simulink model "six_plus_six_AcmsteeringV09_main"  (R2014a)
settings: Solver=FixedStepDiscrete  StartTime=0.0  StopTime=10.0  FixedStep=0.0005  RelTol=1e-3
InitFcn:
  | Veh_Par_wxt
values from neighbouring files (symbols this model uses):
  acc_spdctl = [0 100]    [Veh_Par_wxt.m]
  ag_thr = ecucoder_cal(ag_thr)    [Veh_Par_wxt.m]
  B = 1.8    [Veh_Par_wxt.m]
  bra_em = 100    [Veh_Par_wxt.m]
  bra_pre_gz2 = 100/3    (= 33.3333333333)    [Veh_Par_wxt.m]
  bra_pre_gz34 = 10/3    (= 3.33333333333)    [Veh_Par_wxt.m]
  bra_pre_yd = 10/2    (= 5)    [Veh_Par_wxt.m]
  brakepre_dem_data = [0 1 2 3 4 5 6 7 8 9 10]    [Veh_Par_wxt.m]
  brakeTrq_dem_data = [0 125 251 376 502 627 753 878 1004 1129 1255]    [Veh_Par_wxt.m]
  bratrq_max = 4*1255    (= 5020)    [Veh_Par_wxt.m]
  eff_tran = 0.9    [Veh_Par_wxt.m]
  ESP_switch = ecucoder_cal(ESP_switch)    [Veh_Par_wxt.m]
  G = Mass*g    (= 15696)    [Veh_Par_wxt.m]
  kd1 = ecucoder_cal(kd1)    [Veh_Par_wxt.m]
  kd2 = 0    [Veh_Par_wxt.m]
  ki1 = ecucoder_cal(ki1)    [Veh_Par_wxt.m]
  ki2 = 1    [Veh_Par_wxt.m]
  kp1 = ecucoder_cal(kp1)    [Veh_Par_wxt.m]
  kp2 = 300    [Veh_Par_wxt.m]
  L = L1+L2    (= 2.9)    [Veh_Par_wxt.m]
  premax = 100    [Veh_Par_wxt.m]
  Radius = 0.4572/2    (= 0.2286)    [Veh_Par_wxt.m]
  RC_switch = ecucoder_cal(RC_switch)    [Veh_Par_wxt.m]
  s_opt_yi = 0.15    [Veh_Par_wxt.m]
  s_opt_zhuan = 0.8    [Veh_Par_wxt.m]
  s_opt_zhuan_add = 0.05    [Veh_Par_wxt.m]
  s_opt_zhuan_table = [0.8 0.8 0.3 0.3]    [Veh_Par_wxt.m]
  spd_map_mot = [0 499.85 999.79 1500 2000 2500 3000 3500 4000 4500 4999.8 5999.8]    [Veh_Par_wxt.m]
  spd_spdctl = [0 500]    [Veh_Par_wxt.m]
  speed_thr_park = 5/3.6/Radius*tras_ratio*30/pi    (= 464.143899364)    [Veh_Par_wxt.m]
  TCS_switch = ecucoder_cal(TCS_switch)    [Veh_Par_wxt.m]
  tras_ratio = 8    [Veh_Par_wxt.m]
  trq_map_mot = [70.5 70.012 71.154 65.797 53.917 45.159 38.073 32.685 27.48 17.133 14.949 10.07]    [Veh_Par_wxt.m]
  trqmax_yd = 70.5    [Veh_Par_wxt.m]
  trqmax_zx = 70.5    [Veh_Par_wxt.m]
  trqmaxneg = -70.5    [Veh_Par_wxt.m]
  v_gain = 0.9    [Veh_Par_wxt.m]
  v_table = [0 5 20 100]    [Veh_Par_wxt.m]
  v_thr_park = 5    [Veh_Par_wxt.m]
  zhidong_bianmazhi = [-140000 750000]    [Veh_Par_wxt.m]
  zhidong_down = -140000    [Veh_Par_wxt.m]
  zhidong_up = 750000    [Veh_Par_wxt.m]
  zhidong_youmen = [0 100]    [Veh_Par_wxt.m]
  zhuanxiang_bianmazhi = [-400000 0 400000]    [Veh_Par_wxt.m]
  zhuanxiang_down = -400000    [Veh_Par_wxt.m]
  zhuanxiang_up = 400000    [Veh_Par_wxt.m]
  zhuanxiang_youmen = [-100 0 100]    [Veh_Par_wxt.m]
undefined symbols (not defined in the file or in its folder): ecucoder_acal, guzhang_lf, guzhang_lm, guzhang_lr, guzhang_rf, guzhang_rm, guzhang_rr, myFIS
libraries: simulink x979, ec5744lib x59, fuzblock x2
(part 25 of 26)

== system six_plus_six_AcmsteeringV09_main/MainControl/mode_control/forward/forward/Drive/驱动防滑控制TCS/直行TCS/Subsystem5 ==
  speed_act_rr : Inport
  v_act : Inport  Port=2
  Add : Sum
  Constant : Constant  Value=eps  OutDataTypeStr=single  SampleTime=-1
  Divide : Product  Inputs=*/
  Gain : Gain  Gain=pi/30
  Gain1 : Gain  Gain=Radius
  Gain2 : Gain  Gain=1/3.6
  Gain3 : Gain  Gain=1/tras_ratio
  Subtract : Sum  Inputs=+-
  s_act_rr : Outport
  wires:
  Divide/1 -> s_act_rr/1
  Add/1 -> Divide/2
  Constant/1 -> Add/2
  Subtract/1 -> Divide/1
  Gain1/1 -> Subtract/1, Add/1
  v_act/1 -> Gain2/1
  Gain/1 -> Gain1/1
  speed_act_rr/1 -> Gain3/1
  Gain3/1 -> Gain/1
  Gain2/1 -> Subtract/2

== system six_plus_six_AcmsteeringV09_main/MainControl/mode_control/forward/forward/Drive/驱动防滑控制TCS/直行TCS/Subsystem6 ==
  speed_act_lf : Inport
  speed_act_lm : Inport  Port=2
  speed_act_lr : Inport  Port=3
  Gain : Gain  Gain=1/tras_ratio
  Gain1 : Gain  Gain=pi/30
  Gain2 : Gain  Gain=Radius
  Gain3 : Gain  Gain=3.6
  Gain4 : Gain  Gain=v_gain
  MinMax : MinMax  Inputs=3
  v_act_l : Outport
  wires:
  speed_act_lm/1 -> MinMax/2
  speed_act_lr/1 -> MinMax/3
  speed_act_lf/1 -> MinMax/1
  MinMax/1 -> Gain/1
  Gain/1 -> Gain1/1
  Gain1/1 -> Gain2/1
  Gain2/1 -> Gain3/1
  Gain3/1 -> Gain4/1
  Gain4/1 -> v_act_l/1

== system six_plus_six_AcmsteeringV09_main/MainControl/mode_control/forward/forward/Drive/驱动防滑控制TCS/直行TCS/Subsystem7 ==
  speed_act_rf : Inport
  speed_act_rm : Inport  Port=2
  speed_act_rr : Inport  Port=3
  Gain : Gain  Gain=1/tras_ratio
  Gain1 : Gain  Gain=pi/30
  Gain2 : Gain  Gain=Radius
  Gain3 : Gain  Gain=3.6
  Gain4 : Gain  Gain=v_gain
  MinMax : MinMax  Inputs=3
  v_act_r : Outport
  wires:
  Gain4/1 -> v_act_r/1
  Gain3/1 -> Gain4/1
  Gain2/1 -> Gain3/1
  Gain1/1 -> Gain2/1
  Gain/1 -> Gain1/1
  MinMax/1 -> Gain/1
  speed_act_rf/1 -> MinMax/1
  speed_act_rr/1 -> MinMax/3
  speed_act_rm/1 -> MinMax/2

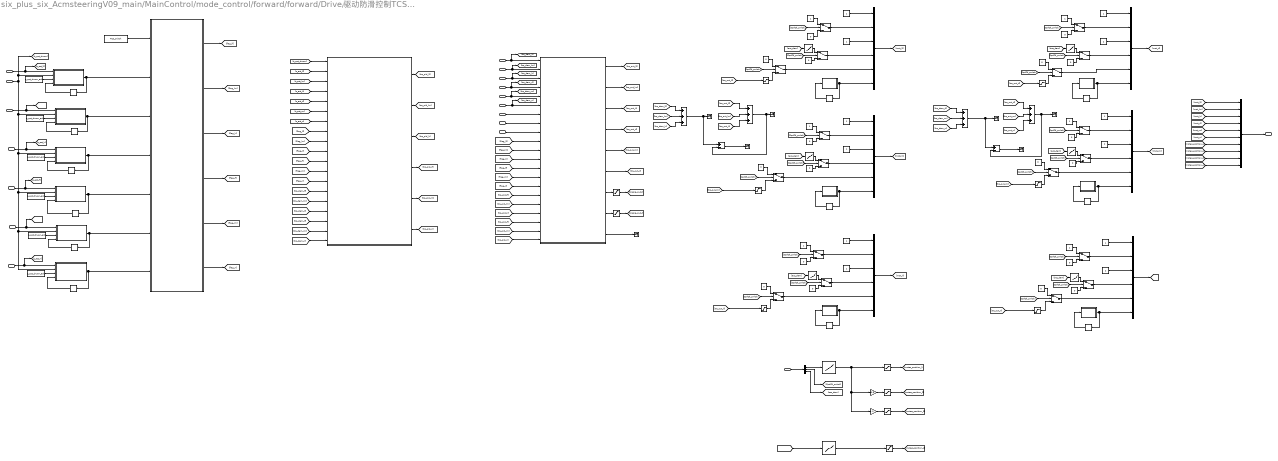
== system six_plus_six_AcmsteeringV09_main/MainControl/mode_control/forward/forward/Drive/驱动防滑控制TCS/直行TCS/直行 ==
  trq_dem_lf : Inport
  trq_dem_lm : Inport  Port=2
  trq_dem_lr : Inport  Port=3
  trq_dem_rf : Inport  Port=4
  trq_dem_rm : Inport  Port=5
  trq_dem_rr : Inport  Port=6
  bra_pre_l : Inport  Port=7
  bra_pre_r : Inport  Port=8
  s_act_lf : Inport  Port=9
  s_act_lm : Inport  Port=10
  s_act_lr : Inport  Port=11
  s_act_rf : Inport  Port=12
  s_act_rm : Inport  Port=13
  s_act_rr : Inport  Port=14
  brake_dem : Inport  Port=15
  s_opt_zhuan : Inport  Port=16
  Signals : Inport  Port=17
  1-D Lookup Table : Lookup_n-D  NumberOfTableDimensions=1  BreakpointsForDimension1=zhuanxiang_youmen  Table=zhuanxiang_bianmazhi  InternalRulePriority=Speed  RndMeth=Simplest  InputSameDT=on
  1-D Lookup Table1 : Lookup_n-D  NumberOfTableDimensions=1  BreakpointsForDimension1=zhidong_youmen  Table=zhidong_bianmazhi  InternalRulePriority=Speed  RndMeth=Simplest  InputSameDT=on
  1-D Lookup Table{2..7} (6 alike) : Lookup_n-D  NumberOfTableDimensions=1  BreakpointsForDimension1=acc_spdctl  Table=spd_spdctl  InternalRulePriority=Speed  RndMeth=Simplest  InputSameDT=on
  Add{,1..3} (4 alike) : Sum  Inputs=+++
  Bus Selector : BusSelector  OutputSignals=RemoteControl_dem.steer_dem,RemoteControl_dem.SpdCtl_switch,RemoteControl_dem.acc_dem
  Constant{,1,3..6} (6 alike) : Constant  Value=0  OutDataTypeStr=single  SampleTime=-1
  Constant{7..10,12..13} (6 alike) : Constant  Value=s_opt_zhuan_add  OutDataTypeStr=single  SampleTime=-1
  Constant11 : Constant  Value=TCS_switch  OutDataTypeStr=single  SampleTime=-1
  Gain : Gain  Gain=0.5
  Gain1 : Gain  Gain=-1
  HeartBeat : MATLAB Function  TreatAsAtomicUnit=on
  HeartBeat1 : MATLAB Function  TreatAsAtomicUnit=on
  HeartBeat2 : MATLAB Function  TreatAsAtomicUnit=on
  HeartBeat3 : MATLAB Function  TreatAsAtomicUnit=on
  HeartBeat4 : MATLAB Function  TreatAsAtomicUnit=on
  HeartBeat5 : MATLAB Function  TreatAsAtomicUnit=on
  MATLAB Function : MATLAB Function  TreatAsAtomicUnit=on
  MATLAB Function1 : MATLAB Function  TreatAsAtomicUnit=on
  MATLAB Function2 : MATLAB Function  TreatAsAtomicUnit=on
  MATLAB Function3 : MATLAB Function  TreatAsAtomicUnit=on
  MATLAB Function4 : MATLAB Function  TreatAsAtomicUnit=on
  MATLAB Function5 : MATLAB Function  TreatAsAtomicUnit=on
  MATLAB Function6 : MATLAB Function  TreatAsAtomicUnit=on
  MATLAB Function7 : MATLAB Function  TreatAsAtomicUnit=on
  Memory{,1..11} (12 alike) : Memory  InheritSampleTime=on
  Mux : Mux  Inputs=10
  Mux{1..6} (6 alike) : Mux  Inputs=6
  Saturation{,1..3,6..7} (6 alike) : Saturate  UpperLimit=trqmax_zx  LowerLimit=trqmaxneg  OutDataTypeStr=single
  Saturation10 : Saturate  UpperLimit=zhuanxiang_up  LowerLimit=zhuanxiang_down
  Saturation11 : Saturate  UpperLimit=zhidong_up  LowerLimit=zhidong_down
  Saturation4 : Saturate  UpperLimit=premax  LowerLimit=0
  Saturation5 : Saturate  UpperLimit=premax  LowerLimit=0
  Saturation8 : Saturate  UpperLimit=zhuanxiang_up  LowerLimit=zhuanxiang_down
  Saturation9 : Saturate  UpperLimit=zhuanxiang_up  LowerLimit=zhuanxiang_down
  SpdSet_dem{,1..5} (6 alike) : Constant  Value=0  OutDataTypeStr=single  SampleTime=-1
  Subsystem : Subsystem
  Subtract : Sum  Inputs=+-
  Subtract1 : Sum  Inputs=+-
  Switch{,1..17} (18 alike) : Switch  Criteria=u2 > Threshold  Threshold=0.5
  Terminator{1..7} (7 alike) : Terminator
  mot_enable{1..6} (6 alike) : Constant  OutDataTypeStr=single  SampleTime=-1
  mot_gear : Constant  OutDataTypeStr=single  SampleTime=-1
  mot_gear1 : Constant  Value=2  OutDataTypeStr=single  SampleTime=-1
  mot_gear2 : Constant  OutDataTypeStr=single  SampleTime=-1
  mot_gear3 : Constant  Value=2  OutDataTypeStr=single  SampleTime=-1
  mot_gear4 : Constant  OutDataTypeStr=single  SampleTime=-1
  mot_gear5 : Constant  Value=2  OutDataTypeStr=single  SampleTime=-1
  mot_mode{,1..5} (6 alike) : Constant  Value=0  OutDataTypeStr=single  SampleTime=-1
  mot_mode{6..11} (6 alike) : Constant  OutDataTypeStr=single  SampleTime=-1
  forward_dem : Outport
  wires:
  Mux/1 -> forward_dem/1
  Memory4/1 -> HeartBeat/1(life_pre)
  HeartBeat/1(life) -> Memory4/1, Mux1/6
  Mux1/1 -> [mot_lf]
  [trq_out_lf] -> Saturation/1  "trq_out_lf_forward"
  mot_gear/1 -> Mux1/3
  mot_enable4/1 -> Mux1/1
  Switch1/1 -> Mux1/4
  Memory1/1 -> HeartBeat2/1(life_pre)
  HeartBeat2/1(life) -> Mux3/6, Memory1/1
  Mux3/1 -> [mot_rf]
  [trq_out_rf] -> Saturation2/1  "trq_out_rf_forward"
  Switch3/1 -> Mux3/2
  mot_gear1/1 -> Mux3/3
  mot_enable2/1 -> Mux3/1
  Switch8/1 -> Mux3/4
  Memory2/1 -> HeartBeat3/1(life_pre)
  HeartBeat3/1(life) -> Mux5/6, Memory2/1
  Mux5/1 -> [mot_lm]
  [trq_out_lm] -> Saturation6/1  "trq_out_lm_forward"
  Switch4/1 -> Mux5/2
  mot_gear2/1 -> Mux5/3
  mot_enable5/1 -> Mux5/1
  Switch10/1 -> Mux5/4
  Memory3/1 -> HeartBeat4/1(life_pre)
  HeartBeat4/1(life) -> Memory3/1, Mux6/6
  Mux6/1 -> [mot_rm]
  [trq_out_rm] -> Saturation7/1  "trq_out_rm_forward"
  Switch5/1 -> Mux6/2
  mot_gear3/1 -> Mux6/3
  mot_enable6/1 -> Mux6/1
  Switch11/1 -> Mux6/4
  Memory5/1 -> HeartBeat1/1(life_pre)
  HeartBeat1/1(life) -> Mux2/6, Memory5/1
  Mux2/1 -> [mot_lr]
  [trq_out_lr] -> Saturation1/1  "trq_out_lr_forward"
  Switch6/1 -> Mux2/2
  mot_gear4/1 -> Mux2/3
  mot_enable1/1 -> Mux2/1
  Switch12/1 -> Mux2/4
  Memory6/1 -> HeartBeat5/1(life_pre)
  HeartBeat5/1(life) -> Memory6/1, Mux4/6
  Mux4/1 -> [mot_rr]
  [trq_out_rr] -> Saturation3/1  "trq_out_rr_forward"
  Switch7/1 -> Mux4/2
  mot_gear5/1 -> Mux4/3
  mot_enable3/1 -> Mux4/1
  Switch13/1 -> Mux4/4
  [mot_lf] -> Mux/1
  [mot_lm] -> Mux/2
  [mot_lr] -> Mux/3
  [mot_rf] -> Mux/4
  [mot_rm] -> Mux/5
  [mot_rr] -> Mux/6
  [motec_position_1] -> Mux/7
  [motec_position_2] -> Mux/8
  [motec_position_3] -> Mux/9
  1-D Lookup Table1/1 -> Saturation11/1
  1-D Lookup Table/1 -> Gain1/1, Gain/1, Saturation8/1
  Signals/1 -> Bus Selector/1
  Gain1/1 -> Saturation10/1
  Bus Selector/1 -> 1-D Lookup Table/1  "<steer_dem>"
  Gain/1 -> Saturation9/1
  Saturation8/1 -> [motec_position_1]
  Saturation9/1 -> [motec_position_2]
  Saturation10/1 -> [motec_position_3]
  Saturation11/1 -> [motec_position_4]
  [brapre_out_l] -> 1-D Lookup Table1/1
  [motec_position_4] -> Mux/10
  Bus Selector/2 -> [SpdCtl_switch]  "<SpdCtl_switch>"
  [SpdCtl_switch] -> Switch/2
  mot_mode6/1 -> Switch/1
  mot_mode/1 -> Switch/3
  Switch/1 -> Mux1/2
  [SpdCtl_switch] -> Switch1/2
  SpdSet_dem/1 -> Switch1/3
  Bus Selector/3 -> [acc_dem]  "<acc_dem>"
  [acc_dem] -> 1-D Lookup Table2/1
  1-D Lookup Table2/1 -> Switch1/1
  [SpdCtl_switch] -> Switch2/2
  Saturation/1 -> Switch2/3
  Constant/1 -> Switch2/1
  Switch2/1 -> Mux1/5
  [SpdCtl_switch] -> Switch3/2
  mot_mode7/1 -> Switch3/1
  mot_mode2/1 -> Switch3/3
  [SpdCtl_switch] -> Switch4/2
  mot_mode8/1 -> Switch4/1
  mot_mode4/1 -> Switch4/3
  [SpdCtl_switch] -> Switch5/2
  mot_mode9/1 -> Switch5/1
  mot_mode5/1 -> Switch5/3
  [SpdCtl_switch] -> Switch6/2
  mot_mode10/1 -> Switch6/1
  mot_mode1/1 -> Switch6/3
  [SpdCtl_switch] -> Switch7/2
  mot_mode11/1 -> Switch7/1
  mot_mode3/1 -> Switch7/3
  [SpdCtl_switch] -> Switch8/2
  [acc_dem] -> 1-D Lookup Table3/1
  1-D Lookup Table3/1 -> Switch8/1
  SpdSet_dem1/1 -> Switch8/3
  [SpdCtl_switch] -> Switch9/2
  Constant1/1 -> Switch9/1
  Saturation2/1 -> Switch9/3
  Switch9/1 -> Mux3/5
  [SpdCtl_switch] -> Switch10/2
  [acc_dem] -> 1-D Lookup Table4/1
  1-D Lookup Table4/1 -> Switch10/1
  SpdSet_dem4/1 -> Switch10/3
  [SpdCtl_switch] -> Switch11/2
  [acc_dem] -> 1-D Lookup Table5/1
  1-D Lookup Table5/1 -> Switch11/1
  SpdSet_dem5/1 -> Switch11/3
  [SpdCtl_switch] -> Switch12/2
  [acc_dem] -> 1-D Lookup Table6/1
  1-D Lookup Table6/1 -> Switch12/1
  SpdSet_dem2/1 -> Switch12/3
  [SpdCtl_switch] -> Switch13/2
  [acc_dem] -> 1-D Lookup Table7/1
  1-D Lookup Table7/1 -> Switch13/1
  SpdSet_dem3/1 -> Switch13/3
  [SpdCtl_switch] -> Switch14/2
  Constant3/1 -> Switch14/1
  Saturation6/1 -> Switch14/3
  Switch14/1 -> Mux5/5
  [SpdCtl_switch] -> Switch15/2
  Constant4/1 -> Switch15/1
  Saturation7/1 -> Switch15/3
  Switch15/1 -> Mux6/5
  [SpdCtl_switch] -> Switch16/2
  Constant5/1 -> Switch16/1
  Saturation1/1 -> Switch16/3
  Switch16/1 -> Mux2/5
  [SpdCtl_switch] -> Switch17/2
  Constant6/1 -> Switch17/1
  Saturation3/1 -> Switch17/3
  Switch17/1 -> Mux4/5
  Constant10/1 -> MATLAB Function3/3(s_opt_zhuan_add)
  Memory9/1 -> MATLAB Function3/4(flag_rr_pre)
  MATLAB Function3/1(flag_rr) -> Memory9/1, MATLAB Function5/7(flag_rr)
  s_act_rr/1 -> [s_act_rr], MATLAB Function3/1(s_act_rr)
  Constant9/1 -> MATLAB Function2/3(s_opt_zhuan_add)
  Memory8/1 -> MATLAB Function2/4(flag_rf_pre)
  MATLAB Function2/1(flag_rf) -> Memory8/1, MATLAB Function5/5(flag_rf)
  s_act_rf/1 -> MATLAB Function2/1(s_act_rf), [s_act_rf]
  Constant8/1 -> MATLAB Function1/3(s_opt_zhuan_add)
  Memory7/1 -> MATLAB Function1/4(flag_lr_pre)
  MATLAB Function1/1(flag_lr) -> Memory7/1, MATLAB Function5/4(flag_lr)
  s_act_lr/1 -> [s_act_lr], MATLAB Function1/1(s_act_lr)
  Constant7/1 -> MATLAB Function/3(s_opt_zhuan_add)
  Memory/1 -> MATLAB Function/4(flag_lf_pre)
  MATLAB Function/1(flag_lf) -> Memory/1, MATLAB Function5/2(flag_lf)
  s_act_lf/1 -> [s_act_lf], MATLAB Function/1(s_act_lf)
  [trq_dem_lf] -> Subsystem/14(trq_dem_lf)
  [flag_lf] -> Subsystem/8(flag_lf)
  [trq_dem_rf] -> Subsystem/17(trq_dem_rf)
  [trq_dem_lr] -> Subsystem/16(trq_dem_lr)
  [flag_lr] -> Subsystem/10(flag_lr)
  [flag_rf] -> Subsystem/11(flag_rf)
  [trq_dem_rr] -> Subsystem/19(trq_dem_rr)
  [flag_rr] -> Subsystem/13(flag_rr)
  [s_opt_zhuan] -> Subsystem/1(s_opt_zhuan)
  [s_act_rr] -> Subsystem/7(s_act_rr)
  [s_act_rf] -> Subsystem/5(s_act_rf)
  [s_act_lr] -> Subsystem/4(s_act_lr)
  [s_act_lf] -> Subsystem/2(s_act_lf)
  Subsystem/3(trq_pid_lr) -> [trq_pid_lr]
  Subsystem/1(trq_pid_lf) -> [trq_pid_lf]
  Subsystem/6(trq_pid_rr) -> [trq_pid_rr]
  Subsystem/4(trq_pid_rf) -> [trq_pid_rf]
  MATLAB Function5/1(flag_lf1) -> [flag_lf]  "flag_lf"
  MATLAB Function5/3(flag_lr1) -> [flag_lr]  "flag_lr"
  MATLAB Function5/4(flag_rf1) -> [flag_rf]  "flag_rf"
  MATLAB Function5/6(flag_rr1) -> [flag_rr]  "flag_rr"
  Constant12/1 -> MATLAB Function4/3(s_opt_zhuan_add)
  Memory10/1 -> MATLAB Function4/4(flag_lm_pre)
  MATLAB Function4/1(flag_lm) -> MATLAB Function5/3(flag_lm), Memory10/1
  s_act_lm/1 -> MATLAB Function4/1(s_act_lm), [s_act_lm]
  Constant13/1 -> MATLAB Function6/3(s_opt_zhuan_add)
  Memory11/1 -> MATLAB Function6/4(flag_rm_pre)
  MATLAB Function6/1(flag_rm) -> Memory11/1, MATLAB Function5/6(flag_rm)
  s_act_rm/1 -> [s_act_rm], MATLAB Function6/1(s_act_rm)
  s_opt_zhuan/1 -> MATLAB Function/2(s_opt_zhuan), [s_opt_zhuan], MATLAB Function4/2(s_opt_zhuan), MATLAB Function1/2(s_opt_zhuan), MATLAB Function2/2(s_opt_zhuan), MATLAB Function6/2(s_opt_zhuan), MATLAB Function3/2(s_opt_zhuan)
  MATLAB Function5/2(flag_lm1) -> [flag_lm]  "flag_lm"
  MATLAB Function5/5(flag_rm1) -> [flag_rm]  "flag_rm"
  Constant11/1 -> MATLAB Function5/1(TCS_switch)
  [s_act_lm] -> Subsystem/3(s_act_lm)
  [s_act_rm] -> Subsystem/6(s_act_rm)
  [flag_lm] -> Subsystem/9(flag_lm)
  [flag_rm] -> Subsystem/12(flag_rm)
  [trq_dem_lm] -> Subsystem/15(trq_dem_lm)
  [trq_dem_rm] -> Subsystem/18(trq_dem_rm)
  Subsystem/2(trq_pid_lm) -> [trq_pid_lm]
  Subsystem/5(trq_pid_rm) -> [trq_pid_rm]
  [flag_rr] -> MATLAB Function7/15(flag_rr)
  [flag_rf] -> MATLAB Function7/13(flag_rf)
  [flag_lr] -> MATLAB Function7/12(flag_lr)
  [flag_lf] -> MATLAB Function7/10(flag_lf)
  [trq_pid_lf] -> MATLAB Function7/16(trq_pid_lf)
  [trq_pid_lr] -> MATLAB Function7/18(trq_pid_lr)
  [trq_pid_rf] -> MATLAB Function7/19(trq_pid_rf)
  [trq_pid_rr] -> MATLAB Function7/21(trq_pid_rr)
  trq_dem_lf/1 -> MATLAB Function7/1(trq_dem_lf), [trq_dem_lf]
  trq_dem_lr/1 -> [trq_dem_lr], MATLAB Function7/3(trq_dem_lr)
  trq_dem_rf/1 -> MATLAB Function7/4(trq_dem_rf), [trq_dem_rf]
  trq_dem_rr/1 -> [trq_dem_rr], MATLAB Function7/6(trq_dem_rr)
  bra_pre_l/1 -> MATLAB Function7/7(bra_pre_l)
  bra_pre_r/1 -> MATLAB Function7/8(bra_pre_r)
  MATLAB Function7/1(trq_out_lf) -> [trq_out_lf]
  MATLAB Function7/3(trq_out_lr) -> [trq_out_lr]
  MATLAB Function7/4(trq_out_rf) -> [trq_out_rf]
  MATLAB Function7/6(trq_out_rr) -> [trq_out_rr]
  MATLAB Function7/7(brapre_out_l) -> Saturation4/1
  MATLAB Function7/8(brapre_out_r) -> Saturation5/1
  brake_dem/1 -> MATLAB Function7/9(brake_dem)
  MATLAB Function7/9(mode) -> Terminator2/1  "TCS_mode"
  Saturation4/1 -> [brapre_out_l]
  Saturation5/1 -> [brapre_out_r]
  MATLAB Function7/2(trq_out_lm) -> [trq_out_lm]
  MATLAB Function7/5(trq_out_rm) -> [trq_out_rm]
  trq_dem_lm/1 -> [trq_dem_lm], MATLAB Function7/2(trq_dem_lm)
  trq_dem_rm/1 -> [trq_dem_rm], MATLAB Function7/5(trq_dem_rm)
  [flag_lm] -> MATLAB Function7/11(flag_lm)
  [flag_rm] -> MATLAB Function7/14(flag_rm)
  [trq_pid_lm] -> MATLAB Function7/17(trq_pid_lm)
  [trq_pid_rm] -> MATLAB Function7/20(trq_pid_rm)
  [trq_out_lm] -> Add/2
  [trq_out_lf] -> Add/1
  [trq_out_lr] -> Add/3
  Add/1 -> Subtract/2, Terminator1/1  "trq_out_l_forward"
  [trq_out_rm] -> Add1/2
  [trq_out_rf] -> Add1/1
  [trq_out_rr] -> Add1/3
  Add1/1 -> Subtract1/2, Terminator3/1  "trq_out_r_forward"
  [trq_dem_lm] -> Add2/2
  [trq_dem_lr] -> Add2/3
  [trq_dem_lf] -> Add2/1
  Add2/1 -> Subtract/1, Terminator4/1  "trq_dem_l_forward"
  Subtract/1 -> Terminator5/1  "trq_adjust_l_forward"
  [trq_dem_rm] -> Add3/2
  [trq_dem_rf] -> Add3/1
  [trq_dem_rr] -> Add3/3
  Add3/1 -> Subtract1/1, Terminator6/1  "trq_dem_r_forward"
  Subtract1/1 -> Terminator7/1  "trq_adjust_r_forward"

== system six_plus_six_AcmsteeringV09_main/MainControl/mode_control/backward/backward/Drive/驱动防滑控制TCS/直行TCS/直行/Subsystem ==
  s_opt_zhuan : Inport
  s_act_lf : Inport  Port=2
  s_act_lm : Inport  Port=3
  s_act_lr : Inport  Port=4
  s_act_rf : Inport  Port=5
  s_act_rm : Inport  Port=6
  s_act_rr : Inport  Port=7
  flag_lf : Inport  Port=8
  flag_lm : Inport  Port=9
  flag_lr : Inport  Port=10
  flag_rf : Inport  Port=11
  flag_rm : Inport  Port=12
  flag_rr : Inport  Port=13
  trq_dem_lf : Inport  Port=14
  trq_dem_lm : Inport  Port=15
  trq_dem_lr : Inport  Port=16
  trq_dem_rf : Inport  Port=17
  trq_dem_rm : Inport  Port=18
  trq_dem_rr : Inport  Port=19
  If{,1..5} (6 alike) : If  IfExpression=u1 > 0.5  ShowElse=off
  Subsystem : Subsystem
  Subsystem1 : Subsystem
  Subsystem2 : Subsystem
  Subsystem3 : Subsystem
  Subsystem4 : Subsystem
  Subsystem5 : Subsystem
  Switch{,1..5} (6 alike) : Switch  Criteria=u2 > Threshold  Threshold=0.5  OutDataTypeStr=single
  trq_pid_lf : Outport
  trq_pid_lm : Outport  Port=2
  trq_pid_lr : Outport  Port=3
  trq_pid_rf : Outport  Port=4
  trq_pid_rm : Outport  Port=5
  trq_pid_rr : Outport  Port=6
  wires:
  Switch/1 -> trq_pid_lf/1
  trq_dem_rr/1 -> Switch2/3, Subsystem3/3(trq_dem_rr)
  flag_rr/1 -> [flag_rr], Switch2/2
  Switch2/1 -> trq_pid_rr/1
  trq_dem_rf/1 -> Subsystem2/3(trq_dem_rf), Switch3/3
  flag_rf/1 -> [flag_rf], Switch3/2
  Switch3/1 -> trq_pid_rf/1
  s_act_lf/1 -> Subsystem/2(s_act_lf)
  Subsystem/1(trq_pid_lf) -> Switch/1
  If/1 -> Subsystem/Action
  flag_lf/1 -> [flag_lf], Switch/2
  trq_dem_lf/1 -> Switch/3, Subsystem/3(trq_dem_lf)
  Switch1/1 -> trq_pid_lr/1
  s_opt_zhuan/1 -> [s_opt_zhuan], Subsystem/1(s_opt_zhuan)
  s_act_lr/1 -> Subsystem1/2(s_act_lr)
  Subsystem1/1(trq_pid_lr) -> Switch1/1
  If1/1 -> Subsystem1/Action
  flag_lr/1 -> [flag_lr], Switch1/2
  trq_dem_lr/1 -> Switch1/3, Subsystem1/3(trq_dem_lr)
  s_act_rf/1 -> Subsystem2/2(s_act_rf)
  Subsystem2/1(trq_pid_rf) -> Switch3/1
  If2/1 -> Subsystem2/Action
  s_act_rr/1 -> Subsystem3/2(s_act_rr)
  Subsystem3/1(trq_pid_rr) -> Switch2/1
  If3/1 -> Subsystem3/Action
  [flag_lf] -> If/1
  [s_opt_zhuan] -> Subsystem2/1(s_opt_zhuan)
  [s_opt_zhuan] -> Subsystem1/1(s_opt_zhuan)
  [s_opt_zhuan] -> Subsystem3/1(s_opt_zhuan)
  [flag_lr] -> If1/1
  [flag_rf] -> If2/1
  Switch4/1 -> trq_pid_lm/1
  s_act_lm/1 -> Subsystem4/2(s_act_lm)
  Subsystem4/1(trq_pid_lm) -> Switch4/1
  If4/1 -> Subsystem4/Action
  flag_lm/1 -> Switch4/2, [flag_lm]
  trq_dem_lm/1 -> Subsystem4/3(trq_dem_lm), Switch4/3
  [s_opt_zhuan] -> Subsystem4/1(s_opt_zhuan)
  [flag_lm] -> If4/1
  trq_dem_rm/1 -> Switch5/3, Subsystem5/3(trq_dem_rm)
  flag_rm/1 -> Switch5/2, [flag_rm]
  Switch5/1 -> trq_pid_rm/1
  s_act_rm/1 -> Subsystem5/2(s_act_rm)
  Subsystem5/1(trq_pid_rm) -> Switch5/1
  If5/1 -> Subsystem5/Action
  [s_opt_zhuan] -> Subsystem5/1(s_opt_zhuan)
  [flag_rm] -> If5/1
  [flag_rr] -> If3/1

== system six_plus_six_AcmsteeringV09_main/MainControl/mode_control/forward/forward/Drive/驱动防滑控制TCS/直行TCS/直行/Subsystem ==
  s_opt_zhuan : Inport
  s_act_lf : Inport  Port=2
  s_act_lm : Inport  Port=3
  s_act_lr : Inport  Port=4
  s_act_rf : Inport  Port=5
  s_act_rm : Inport  Port=6
  s_act_rr : Inport  Port=7
  flag_lf : Inport  Port=8
  flag_lm : Inport  Port=9
  flag_lr : Inport  Port=10
  flag_rf : Inport  Port=11
  flag_rm : Inport  Port=12
  flag_rr : Inport  Port=13
  trq_dem_lf : Inport  Port=14
  trq_dem_lm : Inport  Port=15
  trq_dem_lr : Inport  Port=16
  trq_dem_rf : Inport  Port=17
  trq_dem_rm : Inport  Port=18
  trq_dem_rr : Inport  Port=19
  If{,1..5} (6 alike) : If  IfExpression=u1 > 0.5  ShowElse=off
  Subsystem : Subsystem
  Subsystem1 : Subsystem
  Subsystem2 : Subsystem
  Subsystem3 : Subsystem
  Subsystem4 : Subsystem
  Subsystem5 : Subsystem
  Switch{,1..5} (6 alike) : Switch  Criteria=u2 > Threshold  Threshold=0.5  OutDataTypeStr=single
  trq_pid_lf : Outport
  trq_pid_lm : Outport  Port=2
  trq_pid_lr : Outport  Port=3
  trq_pid_rf : Outport  Port=4
  trq_pid_rm : Outport  Port=5
  trq_pid_rr : Outport  Port=6
  wires:
  Switch/1 -> trq_pid_lf/1
  trq_dem_rr/1 -> Switch2/3, Subsystem3/3(trq_dem_rr)
  flag_rr/1 -> [flag_rr], Switch2/2
  Switch2/1 -> trq_pid_rr/1
  trq_dem_rf/1 -> Subsystem2/3(trq_dem_rf), Switch3/3
  flag_rf/1 -> [flag_rf], Switch3/2
  Switch3/1 -> trq_pid_rf/1
  s_act_lf/1 -> Subsystem/2(s_act_lf)
  Subsystem/1(trq_pid_lf) -> Switch/1
  If/1 -> Subsystem/Action
  flag_lf/1 -> [flag_lf], Switch/2
  trq_dem_lf/1 -> Switch/3, Subsystem/3(trq_dem_lf)
  Switch1/1 -> trq_pid_lr/1
  s_opt_zhuan/1 -> [s_opt_zhuan], Subsystem/1(s_opt_zhuan)
  s_act_lr/1 -> Subsystem1/2(s_act_lr)
  Subsystem1/1(trq_pid_lr) -> Switch1/1
  If1/1 -> Subsystem1/Action
  flag_lr/1 -> [flag_lr], Switch1/2
  trq_dem_lr/1 -> Switch1/3, Subsystem1/3(trq_dem_lr)
  s_act_rf/1 -> Subsystem2/2(s_act_rf)
  Subsystem2/1(trq_pid_rf) -> Switch3/1
  If2/1 -> Subsystem2/Action
  s_act_rr/1 -> Subsystem3/2(s_act_rr)
  Subsystem3/1(trq_pid_rr) -> Switch2/1
  If3/1 -> Subsystem3/Action
  [flag_lf] -> If/1
  [s_opt_zhuan] -> Subsystem2/1(s_opt_zhuan)
  [s_opt_zhuan] -> Subsystem1/1(s_opt_zhuan)
  [s_opt_zhuan] -> Subsystem3/1(s_opt_zhuan)
  [flag_lr] -> If1/1
  [flag_rf] -> If2/1
  Switch4/1 -> trq_pid_lm/1
  s_act_lm/1 -> Subsystem4/2(s_act_lm)
  Subsystem4/1(trq_pid_lm) -> Switch4/1
  If4/1 -> Subsystem4/Action
  flag_lm/1 -> Switch4/2, [flag_lm]
  trq_dem_lm/1 -> Subsystem4/3(trq_dem_lm), Switch4/3
  [s_opt_zhuan] -> Subsystem4/1(s_opt_zhuan)
  [flag_lm] -> If4/1
  trq_dem_rm/1 -> Switch5/3, Subsystem5/3(trq_dem_rm)
  flag_rm/1 -> Switch5/2, [flag_rm]
  Switch5/1 -> trq_pid_rm/1
  s_act_rm/1 -> Subsystem5/2(s_act_rm)
  Subsystem5/1(trq_pid_rm) -> Switch5/1
  If5/1 -> Subsystem5/Action
  [s_opt_zhuan] -> Subsystem5/1(s_opt_zhuan)
  [flag_rm] -> If5/1
  [flag_rr] -> If3/1

== system six_plus_six_AcmsteeringV09_main/MainControl/mode_control/backward/backward/Drive/驱动防滑控制TCS/直行TCS/直行/Subsystem/Subsystem ==
  s_opt_zhuan : Inport
  s_act_lf : Inport  Port=2
  trq_dem_lf : Inport  Port=3
  Action Port : ActionPort  InitializeStates=reset  ActionType=then
  Add10 : Sum  Inputs=+-+
  Add2 : Sum  Inputs=+++
  Add3 : Sum  AccumDataTypeStr=single
  Data Type Conversion : DataTypeConversion
  Gain : Gain  Gain=1/tras_ratio  OutDataTypeStr=Inherit: Inherit via back propagation
  Gain1 : Gain  Gain=kp2  OutDataTypeStr=single
  Gain2 : Gain  Gain=ki2  OutDataTypeStr=single
  Gain20 : Gain  Gain=2
  Gain3 : Gain  Gain=kd2  OutDataTypeStr=single
  Memory{3..5,13} (4 alike) : Memory  InheritSampleTime=on
  Saturation : Saturate  UpperLimit=inf  LowerLimit=0
  Subtract1 : Sum  Inputs=+-
  Subtract5 : Sum
  Sum : Sum  Inputs=|+-
  trq_pid_lf : Outport
  wires:
  trq_dem_lf/1 -> Add3/2
  s_act_lf/1 -> Sum/2
  Add3/1 -> Saturation/1
  Sum/1 -> Subtract1/1, Memory4/1, Add10/1, Gain2/1, Memory3/1
  Gain/1 -> Add3/1
  s_opt_zhuan/1 -> Sum/1
  Gain1/1 -> Add2/1
  Gain2/1 -> Add2/2
  Memory3/1 -> Subtract1/2
  Add10/1 -> Gain3/1
  Gain20/1 -> Add10/2
  Memory5/1 -> Add10/3
  Gain3/1 -> Add2/3
  Subtract1/1 -> Gain1/1
  Memory4/1 -> Memory5/1, Gain20/1
  Add2/1 -> Subtract5/1
  Subtract5/1 -> Memory13/1, Gain/1
  Memory13/1 -> Subtract5/2
  Data Type Conversion/1 -> trq_pid_lf/1
  Saturation/1 -> Data Type Conversion/1

== system six_plus_six_AcmsteeringV09_main/MainControl/mode_control/backward/backward/Drive/驱动防滑控制TCS/直行TCS/直行/Subsystem/Subsystem1 ==
  s_opt_zhuan : Inport
  s_act_lr : Inport  Port=2
  trq_dem_lr : Inport  Port=3
  Action Port : ActionPort  InitializeStates=reset  ActionType=then
  Add10 : Sum  Inputs=+-+
  Add2 : Sum  Inputs=+++
  Add3 : Sum  AccumDataTypeStr=single
  Data Type Conversion : DataTypeConversion
  Gain : Gain  Gain=1/tras_ratio  OutDataTypeStr=Inherit: Inherit via back propagation
  Gain1 : Gain  Gain=kp2  OutDataTypeStr=single
  Gain2 : Gain  Gain=ki2  OutDataTypeStr=single
  Gain20 : Gain  Gain=2
  Gain3 : Gain  Gain=kd2  OutDataTypeStr=single
  Memory{3..5,13} (4 alike) : Memory  InheritSampleTime=on
  Saturation : Saturate  UpperLimit=inf  LowerLimit=0
  Subtract1 : Sum  Inputs=+-
  Subtract5 : Sum
  Sum : Sum  Inputs=|+-
  trq_pid_lr : Outport
  wires:
  trq_dem_lr/1 -> Add3/2
  s_act_lr/1 -> Sum/2
  Add3/1 -> Saturation/1
  Sum/1 -> Subtract1/1, Memory4/1, Add10/1, Gain2/1, Memory3/1
  Gain/1 -> Add3/1
  s_opt_zhuan/1 -> Sum/1
  Gain1/1 -> Add2/1
  Gain2/1 -> Add2/2
  Memory3/1 -> Subtract1/2
  Add10/1 -> Gain3/1
  Gain20/1 -> Add10/2
  Memory5/1 -> Add10/3
  Gain3/1 -> Add2/3
  Subtract1/1 -> Gain1/1
  Memory4/1 -> Memory5/1, Gain20/1
  Add2/1 -> Subtract5/1
  Subtract5/1 -> Gain/1, Memory13/1
  Memory13/1 -> Subtract5/2
  Data Type Conversion/1 -> trq_pid_lr/1
  Saturation/1 -> Data Type Conversion/1

== system six_plus_six_AcmsteeringV09_main/MainControl/mode_control/backward/backward/Drive/驱动防滑控制TCS/直行TCS/直行/Subsystem/Subsystem2 ==
  s_opt_zhuan : Inport
  s_act_rf : Inport  Port=2
  trq_dem_rf : Inport  Port=3
  Action Port : ActionPort  InitializeStates=reset  ActionType=then
  Add11 : Sum  Inputs=+++
  Add8 : Sum  AccumDataTypeStr=single
  Add9 : Sum  Inputs=+-+
  Data Type Conversion2 : DataTypeConversion
  Gain14 : Gain  Gain=1/tras_ratio  OutDataTypeStr=Inherit: Inherit via back propagation
  Gain16 : Gain  Gain=kp2  OutDataTypeStr=single
  Gain17 : Gain  Gain=ki2  OutDataTypeStr=single
  Gain18 : Gain  Gain=2
  Gain19 : Gain  Gain=kd2  OutDataTypeStr=single
  Memory{1..2,6,15} (4 alike) : Memory  InheritSampleTime=on
  Saturation : Saturate  UpperLimit=inf  LowerLimit=0
  Subtract2 : Sum  Inputs=+-
  Subtract7 : Sum
  Sum3 : Sum  Inputs=|+-
  trq_pid_rf : Outport
  wires:
  trq_dem_rf/1 -> Add8/2
  Memory1/1 -> Subtract2/2
  s_act_rf/1 -> Sum3/2
  Subtract2/1 -> Gain16/1
  Add9/1 -> Gain19/1
  Gain17/1 -> Add11/2
  Gain14/1 -> Add8/1
  Gain19/1 -> Add11/3
  Memory6/1 -> Add9/3
  Gain16/1 -> Add11/1
  Add8/1 -> Saturation/1
  s_opt_zhuan/1 -> Sum3/1
  Sum3/1 -> Subtract2/1, Memory2/1, Add9/1, Gain17/1, Memory1/1
  Memory2/1 -> Memory6/1, Gain18/1
  Gain18/1 -> Add9/2
  Memory15/1 -> Subtract7/2
  Add11/1 -> Subtract7/1
  Data Type Conversion2/1 -> trq_pid_rf/1
  Subtract7/1 -> Memory15/1, Gain14/1
  Saturation/1 -> Data Type Conversion2/1

== system six_plus_six_AcmsteeringV09_main/MainControl/mode_control/backward/backward/Drive/驱动防滑控制TCS/直行TCS/直行/Subsystem/Subsystem3 ==
  s_opt_zhuan : Inport
  s_act_rr : Inport  Port=2
  trq_dem_rr : Inport  Port=3
  Action Port : ActionPort  InitializeStates=reset  ActionType=then
  Add12 : Sum  Inputs=+-+
  Add13 : Sum  Inputs=+++
  Add6 : Sum  AccumDataTypeStr=single
  Data Type Conversion3 : DataTypeConversion
  Gain15 : Gain  Gain=1/tras_ratio  OutDataTypeStr=Inherit: Inherit via back propagation
  Gain21 : Gain  Gain=kp2  OutDataTypeStr=single
  Gain22 : Gain  Gain=ki2  OutDataTypeStr=single
  Gain23 : Gain  Gain=2
  Gain24 : Gain  Gain=kd2  OutDataTypeStr=single
  Memory{7..9,16} (4 alike) : Memory  InheritSampleTime=on
  Saturation : Saturate  UpperLimit=inf  LowerLimit=0
  Subtract3 : Sum  Inputs=+-
  Subtract8 : Sum
  Sum2 : Sum  Inputs=|+-
  trq_pid_rr : Outport
  wires:
  trq_dem_rr/1 -> Add6/2
  s_act_rr/1 -> Sum2/2
  Add6/1 -> Saturation/1
  s_opt_zhuan/1 -> Sum2/1
  Sum2/1 -> Memory8/1, Add12/1, Gain22/1, Memory7/1, Subtract3/1
  Gain15/1 -> Add6/1
  Gain21/1 -> Add13/1
  Add13/1 -> Subtract8/1
  Memory8/1 -> Memory9/1, Gain23/1
  Gain23/1 -> Add12/2
  Memory7/1 -> Subtract3/2
  Memory9/1 -> Add12/3
  Data Type Conversion3/1 -> trq_pid_rr/1
  Gain22/1 -> Add13/2
  Add12/1 -> Gain24/1
  Gain24/1 -> Add13/3
  Subtract3/1 -> Gain21/1
  Memory16/1 -> Subtract8/2
  Subtract8/1 -> Gain15/1, Memory16/1
  Saturation/1 -> Data Type Conversion3/1

== system six_plus_six_AcmsteeringV09_main/MainControl/mode_control/backward/backward/Drive/驱动防滑控制TCS/直行TCS/直行/Subsystem/Subsystem4 ==
  s_opt_zhuan : Inport
  s_act_lm : Inport  Port=2
  trq_dem_lm : Inport  Port=3
  Action Port : ActionPort  InitializeStates=reset  ActionType=then
  Add10 : Sum  Inputs=+-+
  Add2 : Sum  Inputs=+++
  Add3 : Sum  AccumDataTypeStr=single
  Data Type Conversion : DataTypeConversion
  Gain : Gain  Gain=1/tras_ratio  OutDataTypeStr=Inherit: Inherit via back propagation
  Gain1 : Gain  Gain=kp2  OutDataTypeStr=single
  Gain2 : Gain  Gain=ki2  OutDataTypeStr=single
  Gain20 : Gain  Gain=2
  Gain3 : Gain  Gain=kd2  OutDataTypeStr=single
  Memory{3..5,13} (4 alike) : Memory  InheritSampleTime=on
  Saturation : Saturate  UpperLimit=inf  LowerLimit=0
  Subtract1 : Sum  Inputs=+-
  Subtract5 : Sum
  Sum : Sum  Inputs=|+-
  trq_pid_lm : Outport
  wires:
  Saturation/1 -> Data Type Conversion/1
  Data Type Conversion/1 -> trq_pid_lm/1
  Memory13/1 -> Subtract5/2
  Subtract5/1 -> Gain/1, Memory13/1
  Add2/1 -> Subtract5/1
  Memory4/1 -> Gain20/1, Memory5/1
  Subtract1/1 -> Gain1/1
  Gain3/1 -> Add2/3
  Memory5/1 -> Add10/3
  Gain20/1 -> Add10/2
  Add10/1 -> Gain3/1
  Memory3/1 -> Subtract1/2
  Gain2/1 -> Add2/2
  Gain1/1 -> Add2/1
  s_opt_zhuan/1 -> Sum/1
  Gain/1 -> Add3/1
  Sum/1 -> Memory3/1, Gain2/1, Add10/1, Memory4/1, Subtract1/1
  Add3/1 -> Saturation/1
  s_act_lm/1 -> Sum/2
  trq_dem_lm/1 -> Add3/2

== system six_plus_six_AcmsteeringV09_main/MainControl/mode_control/backward/backward/Drive/驱动防滑控制TCS/直行TCS/直行/Subsystem/Subsystem5 ==
  s_opt_zhuan : Inport
  s_act_rm : Inport  Port=2
  trq_dem_rm : Inport  Port=3
  Action Port : ActionPort  InitializeStates=reset  ActionType=then
  Add11 : Sum  Inputs=+++
  Add8 : Sum  AccumDataTypeStr=single
  Add9 : Sum  Inputs=+-+
  Data Type Conversion2 : DataTypeConversion
  Gain14 : Gain  Gain=1/tras_ratio  OutDataTypeStr=Inherit: Inherit via back propagation
  Gain16 : Gain  Gain=kp2  OutDataTypeStr=single
  Gain17 : Gain  Gain=ki2  OutDataTypeStr=single
  Gain18 : Gain  Gain=2
  Gain19 : Gain  Gain=kd2  OutDataTypeStr=single
  Memory{1..2,6,15} (4 alike) : Memory  InheritSampleTime=on
  Saturation : Saturate  UpperLimit=inf  LowerLimit=0
  Subtract2 : Sum  Inputs=+-
  Subtract7 : Sum
  Sum3 : Sum  Inputs=|+-
  trq_pid_rm : Outport
  wires:
  Saturation/1 -> Data Type Conversion2/1
  Subtract7/1 -> Gain14/1, Memory15/1
  Data Type Conversion2/1 -> trq_pid_rm/1
  Add11/1 -> Subtract7/1
  Memory15/1 -> Subtract7/2
  Gain18/1 -> Add9/2
  Memory2/1 -> Gain18/1, Memory6/1
  Sum3/1 -> Memory1/1, Gain17/1, Add9/1, Memory2/1, Subtract2/1
  s_opt_zhuan/1 -> Sum3/1
  Add8/1 -> Saturation/1
  Gain16/1 -> Add11/1
  Memory6/1 -> Add9/3
  Gain19/1 -> Add11/3
  Gain14/1 -> Add8/1
  Gain17/1 -> Add11/2
  Add9/1 -> Gain19/1
  Subtract2/1 -> Gain16/1
  s_act_rm/1 -> Sum3/2
  Memory1/1 -> Subtract2/2
  trq_dem_rm/1 -> Add8/2

== system six_plus_six_AcmsteeringV09_main/MainControl/mode_control/forward/forward/Drive/驱动防滑控制TCS/直行TCS/直行/Subsystem/Subsystem ==
  s_opt_zhuan : Inport
  s_act_lf : Inport  Port=2
  trq_dem_lf : Inport  Port=3
  Action Port : ActionPort  InitializeStates=reset  ActionType=then
  Add10 : Sum  Inputs=+-+
  Add2 : Sum  Inputs=+++
  Add3 : Sum  AccumDataTypeStr=single
  Data Type Conversion : DataTypeConversion
  Gain : Gain  Gain=1/tras_ratio  OutDataTypeStr=Inherit: Inherit via back propagation
  Gain1 : Gain  Gain=kp2  OutDataTypeStr=single
  Gain2 : Gain  Gain=ki2  OutDataTypeStr=single
  Gain20 : Gain  Gain=2
  Gain3 : Gain  Gain=kd2  OutDataTypeStr=single
  Memory{3..5,13} (4 alike) : Memory  InheritSampleTime=on
  Saturation : Saturate  UpperLimit=inf  LowerLimit=0
  Subtract1 : Sum  Inputs=+-
  Subtract5 : Sum
  Sum : Sum  Inputs=|+-
  trq_pid_lf : Outport
  wires:
  trq_dem_lf/1 -> Add3/2
  s_act_lf/1 -> Sum/2
  Add3/1 -> Saturation/1
  Sum/1 -> Subtract1/1, Memory4/1, Add10/1, Gain2/1, Memory3/1
  Gain/1 -> Add3/1  "trq_pid_lf_adjust"
  s_opt_zhuan/1 -> Sum/1
  Gain1/1 -> Add2/1
  Gain2/1 -> Add2/2
  Memory3/1 -> Subtract1/2
  Add10/1 -> Gain3/1
  Gain20/1 -> Add10/2
  Memory5/1 -> Add10/3
  Gain3/1 -> Add2/3
  Subtract1/1 -> Gain1/1
  Memory4/1 -> Memory5/1, Gain20/1
  Add2/1 -> Subtract5/1
  Subtract5/1 -> Memory13/1, Gain/1
  Memory13/1 -> Subtract5/2
  Data Type Conversion/1 -> trq_pid_lf/1
  Saturation/1 -> Data Type Conversion/1

== system six_plus_six_AcmsteeringV09_main/MainControl/mode_control/forward/forward/Drive/驱动防滑控制TCS/直行TCS/直行/Subsystem/Subsystem1 ==
  s_opt_zhuan : Inport
  s_act_lr : Inport  Port=2
  trq_dem_lr : Inport  Port=3
  Action Port : ActionPort  InitializeStates=reset  ActionType=then
  Add10 : Sum  Inputs=+-+
  Add2 : Sum  Inputs=+++
  Add3 : Sum  AccumDataTypeStr=single
  Data Type Conversion : DataTypeConversion
  Gain : Gain  Gain=1/tras_ratio  OutDataTypeStr=Inherit: Inherit via back propagation
  Gain1 : Gain  Gain=kp2  OutDataTypeStr=single
  Gain2 : Gain  Gain=ki2  OutDataTypeStr=single
  Gain20 : Gain  Gain=2
  Gain3 : Gain  Gain=kd2  OutDataTypeStr=single
  Memory{3..5,13} (4 alike) : Memory  InheritSampleTime=on
  Saturation : Saturate  UpperLimit=inf  LowerLimit=0
  Subtract1 : Sum  Inputs=+-
  Subtract5 : Sum
  Sum : Sum  Inputs=|+-
  trq_pid_lr : Outport
  wires:
  trq_dem_lr/1 -> Add3/2
  s_act_lr/1 -> Sum/2
  Add3/1 -> Saturation/1
  Sum/1 -> Subtract1/1, Memory4/1, Add10/1, Gain2/1, Memory3/1
  Gain/1 -> Add3/1  "trq_pid_lr_adjust"
  s_opt_zhuan/1 -> Sum/1
  Gain1/1 -> Add2/1
  Gain2/1 -> Add2/2
  Memory3/1 -> Subtract1/2
  Add10/1 -> Gain3/1
  Gain20/1 -> Add10/2
  Memory5/1 -> Add10/3
  Gain3/1 -> Add2/3
  Subtract1/1 -> Gain1/1
  Memory4/1 -> Memory5/1, Gain20/1
  Add2/1 -> Subtract5/1
  Subtract5/1 -> Gain/1, Memory13/1
  Memory13/1 -> Subtract5/2
  Data Type Conversion/1 -> trq_pid_lr/1
  Saturation/1 -> Data Type Conversion/1

== system six_plus_six_AcmsteeringV09_main/MainControl/mode_control/forward/forward/Drive/驱动防滑控制TCS/直行TCS/直行/Subsystem/Subsystem2 ==
  s_opt_zhuan : Inport
  s_act_rf : Inport  Port=2
  trq_dem_rf : Inport  Port=3
  Action Port : ActionPort  InitializeStates=reset  ActionType=then
  Add11 : Sum  Inputs=+++
  Add8 : Sum  AccumDataTypeStr=single
  Add9 : Sum  Inputs=+-+
  Data Type Conversion2 : DataTypeConversion
  Gain14 : Gain  Gain=1/tras_ratio  OutDataTypeStr=Inherit: Inherit via back propagation
  Gain16 : Gain  Gain=kp2  OutDataTypeStr=single
  Gain17 : Gain  Gain=ki2  OutDataTypeStr=single
  Gain18 : Gain  Gain=2
  Gain19 : Gain  Gain=kd2  OutDataTypeStr=single
  Memory{1..2,6,15} (4 alike) : Memory  InheritSampleTime=on
  Saturation : Saturate  UpperLimit=inf  LowerLimit=0
  Subtract2 : Sum  Inputs=+-
  Subtract7 : Sum
  Sum3 : Sum  Inputs=|+-
  trq_pid_rf : Outport
  wires:
  trq_dem_rf/1 -> Add8/2
  Memory1/1 -> Subtract2/2
  s_act_rf/1 -> Sum3/2
  Subtract2/1 -> Gain16/1
  Add9/1 -> Gain19/1
  Gain17/1 -> Add11/2
  Gain14/1 -> Add8/1  "trq_pid_rf_adjust"
  Gain19/1 -> Add11/3
  Memory6/1 -> Add9/3
  Gain16/1 -> Add11/1
  Add8/1 -> Saturation/1
  s_opt_zhuan/1 -> Sum3/1
  Sum3/1 -> Subtract2/1, Memory2/1, Add9/1, Gain17/1, Memory1/1
  Memory2/1 -> Memory6/1, Gain18/1
  Gain18/1 -> Add9/2
  Memory15/1 -> Subtract7/2
  Add11/1 -> Subtract7/1
  Data Type Conversion2/1 -> trq_pid_rf/1
  Subtract7/1 -> Memory15/1, Gain14/1
  Saturation/1 -> Data Type Conversion2/1

== system six_plus_six_AcmsteeringV09_main/MainControl/mode_control/forward/forward/Drive/驱动防滑控制TCS/直行TCS/直行/Subsystem/Subsystem3 ==
  s_opt_zhuan : Inport
  s_act_rr : Inport  Port=2
  trq_dem_rr : Inport  Port=3
  Action Port : ActionPort  InitializeStates=reset  ActionType=then
  Add12 : Sum  Inputs=+-+
  Add13 : Sum  Inputs=+++
  Add6 : Sum  AccumDataTypeStr=single
  Data Type Conversion3 : DataTypeConversion
  Gain15 : Gain  Gain=1/tras_ratio  OutDataTypeStr=Inherit: Inherit via back propagation
  Gain21 : Gain  Gain=kp2  OutDataTypeStr=single
  Gain22 : Gain  Gain=ki2  OutDataTypeStr=single
  Gain23 : Gain  Gain=2
  Gain24 : Gain  Gain=kd2  OutDataTypeStr=single
  Memory{7..9,16} (4 alike) : Memory  InheritSampleTime=on
  Saturation : Saturate  UpperLimit=inf  LowerLimit=0
  Subtract3 : Sum  Inputs=+-
  Subtract8 : Sum
  Sum2 : Sum  Inputs=|+-
  trq_pid_rr : Outport
  wires:
  trq_dem_rr/1 -> Add6/2
  s_act_rr/1 -> Sum2/2
  Add6/1 -> Saturation/1
  s_opt_zhuan/1 -> Sum2/1
  Sum2/1 -> Memory8/1, Add12/1, Gain22/1, Memory7/1, Subtract3/1
  Gain15/1 -> Add6/1  "trq_pid_rr_adjust"
  Gain21/1 -> Add13/1
  Add13/1 -> Subtract8/1
  Memory8/1 -> Memory9/1, Gain23/1
  Gain23/1 -> Add12/2
  Memory7/1 -> Subtract3/2
  Memory9/1 -> Add12/3
  Data Type Conversion3/1 -> trq_pid_rr/1
  Gain22/1 -> Add13/2
  Add12/1 -> Gain24/1
  Gain24/1 -> Add13/3
  Subtract3/1 -> Gain21/1
  Memory16/1 -> Subtract8/2
  Subtract8/1 -> Gain15/1, Memory16/1
  Saturation/1 -> Data Type Conversion3/1

== system six_plus_six_AcmsteeringV09_main/MainControl/mode_control/forward/forward/Drive/驱动防滑控制TCS/直行TCS/直行/Subsystem/Subsystem4 ==
  s_opt_zhuan : Inport
  s_act_lm : Inport  Port=2
  trq_dem_lm : Inport  Port=3
  Action Port : ActionPort  InitializeStates=reset  ActionType=then
  Add10 : Sum  Inputs=+-+
  Add2 : Sum  Inputs=+++
  Add3 : Sum  AccumDataTypeStr=single
  Data Type Conversion : DataTypeConversion
  Gain : Gain  Gain=1/tras_ratio  OutDataTypeStr=Inherit: Inherit via back propagation
  Gain1 : Gain  Gain=kp2  OutDataTypeStr=single
  Gain2 : Gain  Gain=ki2  OutDataTypeStr=single
  Gain20 : Gain  Gain=2
  Gain3 : Gain  Gain=kd2  OutDataTypeStr=single
  Memory{3..5,13} (4 alike) : Memory  InheritSampleTime=on
  Saturation : Saturate  UpperLimit=inf  LowerLimit=0
  Subtract1 : Sum  Inputs=+-
  Subtract5 : Sum
  Sum : Sum  Inputs=|+-
  trq_pid_lm : Outport
  wires:
  Saturation/1 -> Data Type Conversion/1
  Data Type Conversion/1 -> trq_pid_lm/1
  Memory13/1 -> Subtract5/2
  Subtract5/1 -> Gain/1, Memory13/1
  Add2/1 -> Subtract5/1
  Memory4/1 -> Gain20/1, Memory5/1
  Subtract1/1 -> Gain1/1
  Gain3/1 -> Add2/3
  Memory5/1 -> Add10/3
  Gain20/1 -> Add10/2
  Add10/1 -> Gain3/1
  Memory3/1 -> Subtract1/2
  Gain2/1 -> Add2/2
  Gain1/1 -> Add2/1
  s_opt_zhuan/1 -> Sum/1
  Gain/1 -> Add3/1  "trq_pid_lm_adjust"
  Sum/1 -> Memory3/1, Gain2/1, Add10/1, Memory4/1, Subtract1/1
  Add3/1 -> Saturation/1
  s_act_lm/1 -> Sum/2
  trq_dem_lm/1 -> Add3/2

== system six_plus_six_AcmsteeringV09_main/MainControl/mode_control/forward/forward/Drive/驱动防滑控制TCS/直行TCS/直行/Subsystem/Subsystem5 ==
  s_opt_zhuan : Inport
  s_act_rm : Inport  Port=2
  trq_dem_rm : Inport  Port=3
  Action Port : ActionPort  InitializeStates=reset  ActionType=then
  Add11 : Sum  Inputs=+++
  Add8 : Sum  AccumDataTypeStr=single
  Add9 : Sum  Inputs=+-+
  Data Type Conversion2 : DataTypeConversion
  Gain14 : Gain  Gain=1/tras_ratio  OutDataTypeStr=Inherit: Inherit via back propagation
  Gain16 : Gain  Gain=kp2  OutDataTypeStr=single
  Gain17 : Gain  Gain=ki2  OutDataTypeStr=single
  Gain18 : Gain  Gain=2
  Gain19 : Gain  Gain=kd2  OutDataTypeStr=single
  Memory{1..2,6,15} (4 alike) : Memory  InheritSampleTime=on
  Saturation : Saturate  UpperLimit=inf  LowerLimit=0
  Subtract2 : Sum  Inputs=+-
  Subtract7 : Sum
  Sum3 : Sum  Inputs=|+-
  trq_pid_rm : Outport
  wires:
  Saturation/1 -> Data Type Conversion2/1
  Subtract7/1 -> Gain14/1, Memory15/1
  Data Type Conversion2/1 -> trq_pid_rm/1
  Add11/1 -> Subtract7/1
  Memory15/1 -> Subtract7/2
  Gain18/1 -> Add9/2
  Memory2/1 -> Gain18/1, Memory6/1
  Sum3/1 -> Memory1/1, Gain17/1, Add9/1, Memory2/1, Subtract2/1
  s_opt_zhuan/1 -> Sum3/1
  Add8/1 -> Saturation/1
  Gain16/1 -> Add11/1
  Memory6/1 -> Add9/3
  Gain19/1 -> Add11/3
  Gain14/1 -> Add8/1  "trq_pid_rm_adjust"
  Gain17/1 -> Add11/2
  Add9/1 -> Gain19/1
  Subtract2/1 -> Gain16/1
  s_act_rm/1 -> Sum3/2
  Memory1/1 -> Subtract2/2
  trq_dem_rm/1 -> Add8/2

== matlab function six_plus_six_AcmsteeringV09_main/MainControl/mode_control/Park/park/HeartBeat ==
  data: life_pre input; life output
function life = fcn(life_pre)
%#codegen
life=single(life_pre+1);
if life>255
    life=single(0);
end
end

== matlab function six_plus_six_AcmsteeringV09_main/MainControl/mode_control/forward/forward/Drive/目标转向力矩确定模块/MATLAB Function2 ==
  data: umax input; delta_Tsteer_max output; G input; L input; B input; Radius input; Rturn_min_xy input
function delta_Tsteer_max = fcn(umax,G,L,B,Radius,Rturn_min_xy)
%#codegen

    delta_Fsteer_max=single(umax/(0.925+0.15*(Rturn_min_xy/B))*G*L/(2*B));
    delta_Tsteer_max=single(delta_Fsteer_max*Radius);
    
end

== matlab function six_plus_six_AcmsteeringV09_main/MainControl/mode_control/Park/park/HeartBeat1 ==
  data: life_pre input; life output
function life = fcn(life_pre)
%#codegen
life=single(life_pre+1);
if life>255
    life=single(0);
end
end

== matlab function six_plus_six_AcmsteeringV09_main/MainControl/mode_control/forward/forward/Drive/目标转向力矩确定模块/MATLAB Function ==
  data: steer_dem input; Rturn_min output; G input; L input; umax input; B input; Tpeak_L input; Tpeak_R input; eff_tran input; Radius input; f input
function Rturn_min = fcn(steer_dem,G,L,umax,B,Tpeak_L,Tpeak_R,eff_tran,Radius,f)
%#codegen
if steer_dem>0
    Rturn_min=single((G*L*umax/(4*B*(Tpeak_R*eff_tran/Radius-f*G/2))-0.925)/0.15*B);
else
    Rturn_min=single((G*L*umax/(4*B*(Tpeak_L*eff_tran/Radius-f*G/2))-0.925)/0.15*B);
end
end

== matlab function six_plus_six_AcmsteeringV09_main/MainControl/mode_control/forward/forward/Drive/目标转向力矩确定模块/MATLAB Function1 ==
  data: v_act input; Rturn_min_ag output; ag_thr input
 function Rturn_min_ag = fcn(v_act,ag_thr)
%#codegen

    Rturn_min_ag=single((v_act/3.6)^2/ag_thr);
end

== matlab function six_plus_six_AcmsteeringV09_main/Data_input/181/Enabled
Subsystem/MATLAB Function3 ==
  data: speed input; speed_out output
function speed_out = motec_speed(speed)
    if speed>32768
        speed_out=speed-65535;
    else speed_out=speed;
    end
end

== matlab function six_plus_six_AcmsteeringV09_main/MainControl/mode_control/forward/forward/Drive/驱动防滑控制TCS/直行TCS/直行/HeartBeat2 ==
  data: life_pre input; life output
function life = fcn(life_pre)
%#codegen
life=single(life_pre+1);
if life>255
    life=single(0);
end
end

== matlab function six_plus_six_AcmsteeringV09_main/MainControl/mode_control/forward/forward/Drive/左右侧电机分配及功率限制/MATLAB Function ==
  data: trqlim_l input; trq_dem_l output; trq_dem_r output; trq_dem_l1 input; trqlim_r input; trq_dem_r1 input; delta_T_dem input
function [trq_dem_l,trq_dem_r] = fcn(trqlim_l,trq_dem_l1,trqlim_r,trq_dem_r1,delta_T_dem)
%#codegen
if trq_dem_l1==trqlim_l
    trq_dem_l=single(trq_dem_l1);
    trq_dem_r=single(trq_dem_l1+delta_T_dem);%这时候加的是负值
elseif trq_dem_r1==trqlim_r
    trq_dem_l=single(trq_dem_r1-delta_T_dem);
    trq_dem_r=single(trq_dem_r1);
    
else
    trq_dem_l=single(trq_dem_l1);
    trq_dem_r=single(trq_dem_r1);
end
% trq_dem_l=single(max(0,trq_dem_l));%限一下最小值，不要小于0
% trq_dem_r=single(max(0,trq_dem_r));
trq_dem_l=single(max(-trqlim_l,trq_dem_l));%小转向半径下，内侧履带是可能输出负转矩的，从地面吸收功率，给外侧，所以不能限到0，限到最大电机外特性负值
trq_dem_r=single(max(-trqlim_r,trq_dem_r));
end
